simulink model "motor"  (R2020b)
settings: Solver=FixedStepAuto  StartTime=0.0  StopTime=10  FixedStep=0.001  RelTol=1e-3
undefined symbols (not defined in the file or in its folder): k1, k2
settings Model: Creator=lqy  LastModifiedBy=96919
settings DataIOCC: ReturnWorkspaceOutputs=off
settings DebuggingCC: ArithmeticOperatorsInVariantConditions=warning
settings SFSimCC: SimUseLocalCustomCode=off  CustomCodeUndefinedFunction=UseInterfaceOnly
settings RTWCC: RTWUseLocalCustomCode=off
settings CodeAppCC: StateflowObjectComments=on

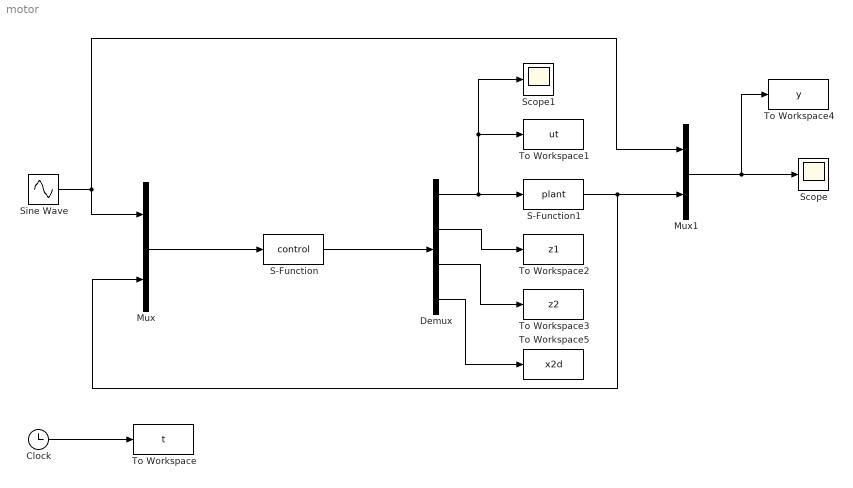
== system motor ==
  Clock : Clock
  Demux : Demux
  Mux : Mux  Inputs=2
  Mux1 : Mux  Inputs=2
  S-Function : S-Function  FunctionName=control  Parameters=k1,k2  SFunctionDeploymentMode=off  EnableBusSupport=off
  S-Function1 : S-Function  FunctionName=plant  SFunctionDeploymentMode=off  EnableBusSupport=off
  Scope : Scope
  Scope1 : Scope
  Sine Wave : Sin  SampleTime=0
  To Workspace : ToWorkspace  VariableName=t  SampleTime=-1
  To Workspace1 : ToWorkspace  VariableName=ut  SampleTime=-1
  To Workspace2 : ToWorkspace  VariableName=z1  SampleTime=-1
  To Workspace3 : ToWorkspace  VariableName=z2  SampleTime=-1
  To Workspace4 : ToWorkspace  VariableName=y  SampleTime=-1
  To Workspace5 : ToWorkspace  VariableName=x2d  SampleTime=-1
  wires:
  Sine Wave/1 -> Mux/1, Mux1/1
  S-Function1/1 -> Mux1/2, Mux/2
  S-Function/1 -> Demux/1
  Demux/1 -> Scope1/1, To Workspace1/1, S-Function1/1
  Clock/1 -> To Workspace/1
  Mux1/1 -> To Workspace4/1, Scope/1
  Demux/2 -> To Workspace2/1
  Demux/3 -> To Workspace3/1
  Demux/4 -> To Workspace5/1
  Mux/1 -> S-Function/1
